simulink model "Senorless"  (R2023a)
settings: Solver=FixedStepDiscrete  StartTime=0.0  StopTime=5  FixedStep=1/FOC_FRQ  RelTol=1e-3
values from neighbouring files (symbols this model uses):
  ADC_REF = 3.6    [Senorless.sldd]
  ADC_SAMPLE_MAX = 32767.0    [Senorless.sldd]
  AMP_GAIN = 16.0    [Senorless.sldd]
  CURR_INPUT = 3276.0    [Senorless.sldd]
  CURR_KI = 380.0    [Senorless.sldd]
  CURR_KP = 0.04    [Senorless.sldd]
  CURR_LIMIT = 0.95    [Senorless.sldd]
  CURR_OVER = 6.0    [Senorless.sldd]
  CURR_POINT_GAIN = 7.0    [Senorless.sldd]
  CURR_STEP = 32760.0    [Senorless.sldd]
  CURR_UNDER = 0.03    [Senorless.sldd]
  CURR_WIDTH = 6552.0    [Senorless.sldd]
  FOC_FRQ = 25000.0    [Senorless.sldd]
  GAMMA = 32767.0    [Senorless.sldd]
  IMAX = 10.0    [Senorless.sldd]
  LPF_FRQ = 2000.0    [Senorless.sldd]
  MOTOR_DAMPER = 2.06E-7    [Senorless.sldd]
  MOTOR_FLUX = 0.00212352    [Senorless.sldd]
  MOTOR_INERTIA = 4.0E-7    [Senorless.sldd]
  MOTOR_LS = 0.000536    [Senorless.sldd]
  MOTOR_PN = 7.0    [Senorless.sldd]
  MOTOR_RS = 4.0    [Senorless.sldd]
  OPEN_IQ = 0.28    [Senorless.sldd]
  OPEN_IQ_MIN = 0.05    [Senorless.sldd]
  OPEN_IQ_SLOW = 0.1    [Senorless.sldd]
  OPEN_SPD = 1000.0    [Senorless.sldd]
  OPEN_SPD_SLOW = 180.0    [Senorless.sldd]
  OPEN_TIME = 0.5    [Senorless.sldd]
  OPEN_TIME_NFO = 0.5    [Senorless.sldd]
  PLL_LIMIT = 0.9    [Senorless.sldd]
  PLL_WIDTH = 800.0    [Senorless.sldd]
  PWM_FRQ = 96000000.0    [Senorless.sldd]
  RS_HUNT = 0.02    [Senorless.sldd]
  SMOK_FRQ = 600.0    [Senorless.sldd]
  SPD_LIMIT = 0.9    [Senorless.sldd]
  SPD_LPF_LEVEL = 0.0    [Senorless.sldd]
  SPD_MAX = 12000.0    [Senorless.sldd]
  SPD_MIN = 4000.0    [Senorless.sldd]
  SPD_REDUCE = 380.0    [Senorless.sldd]
  SPD_STEP = 6.0    [Senorless.sldd]
  SPD_WIDTH = 20.0    [Senorless.sldd]
  THETA_ERR_LIMIT = 8192.0    [Senorless.sldd]
  TS_POINT_GAIN = 10.0    [Senorless.sldd]
  UDC = 48.0    [Senorless.sldd]
  UDC_GAIN = 21.0    [Senorless.sldd]
  UDC_POINT_GAIN = 10.0    [Senorless.sldd]
undefined symbols (not defined in the file or in its folder): curr_q_ki, curr_q_kp, DiscIntNeverNeededParam, magnitude, PLL_LPF_LEVEL, Udc
libraries: simulink x20, slpidlib x5, mcbcontrolslib x2, mcbplantlib x1, autolibpmsmexterior x1, spspowerguiLib x1
(part 2 of 8)

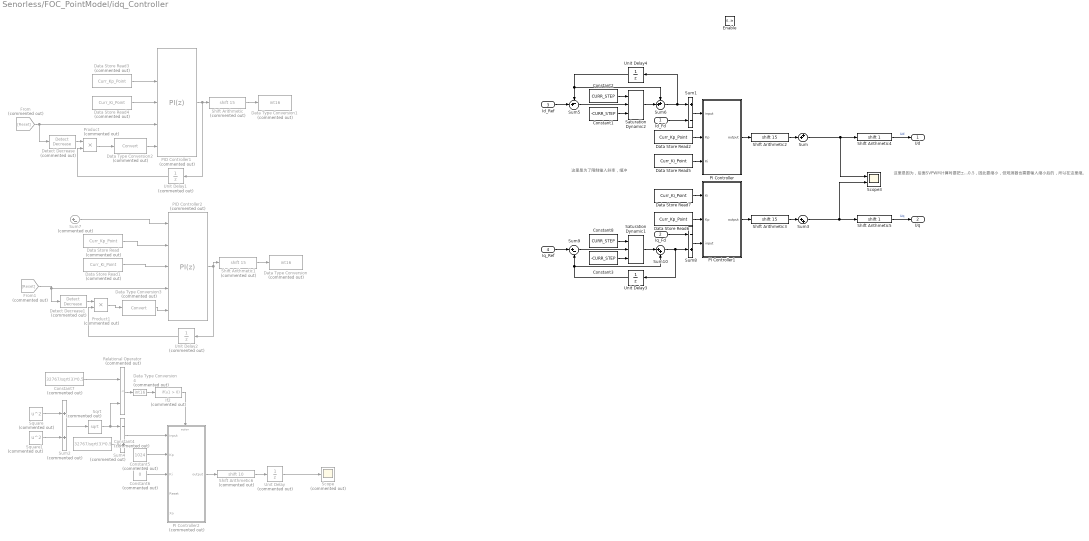
== system Senorless/FOC_PointModel/idq_Controller ==
  note: 这里是为了限制输入斜率，缓冲
  note: 这里是因为，后面SVPWM计算时要把±1映射去±0.5，因此要缩小，但观测器也需要输入缩小后的，所以在这里缩。
  Id_Fd : Inport
  Iq_Fd : Inport  Port=2
  Id_Ref : Inport  Port=3
  Iq_Ref : Inport  Port=4
  Enable : EnablePort  StatesWhenEnabling=reset
  Constant1 : Constant  Value=-CURR_STEP  OutDataTypeStr=int16
  Constant2 : Constant  Value=CURR_STEP  OutDataTypeStr=int16
  Constant3 : Constant  Value=-CURR_STEP  OutDataTypeStr=int16
  Constant4 : Constant  Commented=on  Value=32767/sqrt(3)*0.5  OutDataTypeStr=int32
  Constant5 : Constant  Commented=on  Value=1024  OutDataTypeStr=int16
  Constant6 : Constant  Commented=on  Value=0  OutDataTypeStr=int16
  Constant7 : Constant  Commented=on  Value=32767/sqrt(3)*0.5  OutDataTypeStr=int32
  Constant8 : Constant  Value=CURR_STEP  OutDataTypeStr=int16
  Data Store Read : DataStoreRead  Commented=on  DataStoreName=Curr_Kp_Point  IndexOptions=Index vector (dialog)  Indices=1  OutputSizes=1
  Data Store Read1 : DataStoreRead  Commented=on  DataStoreName=Curr_Ki_Point  IndexOptions=Index vector (dialog)  Indices=1  OutputSizes=1
  Data Store Read2 : DataStoreRead  DataStoreName=Curr_Kp_Point  IndexOptions=Index vector (dialog)  Indices=1  OutputSizes=1
  Data Store Read3 : DataStoreRead  Commented=on  DataStoreName=Curr_Kp_Point  IndexOptions=Index vector (dialog)  Indices=1  OutputSizes=1
  Data Store Read4 : DataStoreRead  Commented=on  DataStoreName=Curr_Ki_Point  IndexOptions=Index vector (dialog)  Indices=1  OutputSizes=1
  Data Store Read5 : DataStoreRead  DataStoreName=Curr_Ki_Point  IndexOptions=Index vector (dialog)  Indices=1  OutputSizes=1
  Data Store Read6 : DataStoreRead  DataStoreName=Curr_Kp_Point  IndexOptions=Index vector (dialog)  Indices=1  OutputSizes=1
  Data Store Read7 : DataStoreRead  DataStoreName=Curr_Ki_Point  IndexOptions=Index vector (dialog)  Indices=1  OutputSizes=1
  Data Type Conversion : DataTypeConversion  Commented=on  OutDataTypeStr=int16  SaturateOnIntegerOverflow=off  RndMeth=Floor
  Data Type Conversion1 : DataTypeConversion  Commented=on  OutDataTypeStr=int16  SaturateOnIntegerOverflow=off  RndMeth=Floor
  Data Type Conversion2 : DataTypeConversion  Commented=on  SaturateOnIntegerOverflow=off  RndMeth=Floor
  Data Type Conversion3 : DataTypeConversion  Commented=on  SaturateOnIntegerOverflow=off  RndMeth=Floor
  Data Type Conversion4 : DataTypeConversion  Commented=on  OutDataTypeStr=int16  SaturateOnIntegerOverflow=off
  Detect Decrease : simulink/Logic and Bit Operations/Detect Decrease  Commented=on  vinit=0.0  OutDataTypeStr=uint8
  Detect Decrease1 : simulink/Logic and Bit Operations/Detect Decrease  Commented=on  vinit=0.0  OutDataTypeStr=uint8
  From : From  Commented=on  GotoTag=Reset
  From1 : From  Commented=on  GotoTag=Reset
  If2 : If  Commented=on  ShowElse=off
  PI Controller : Subsystem
      settings: MinAlgLoopOccurrences=on
  PI Controller1 : Subsystem
      settings: MinAlgLoopOccurrences=on
  PI Controller2 : Subsystem  Commented=on  TreatAsAtomicUnit=on
      settings: MinAlgLoopOccurrences=on
  PID Controller1 : slpidlib/PID Controller  Commented=on  Controller=PI  Form=Parallel  TimeDomain=Discrete-time  UseExternalTs=off  SampleTime=-1  IntegratorMethod=Forward Euler  FilterMethod=Forward Euler  ControllerParametersSource=external  P=curr_q_kp  I=curr_q_ki  UseKiTs=off  D=0  N=100  UseFilter=on  TunerSelectOption=Transfer Function Based (PID Tuner App)  ZeroCross=off  InitialConditionSource=external  InitialConditionForIntegrator=0  InitialConditionForFilter=0  DifferentiatorICPrevScaledInput=0  ExternalReset=either  TrackingMode=off  Kt=1  LimitOutput=on  SatLimitsSource=internal  UpperSaturationLimit=32767*32767  LowerSaturationLimit=-32767*32767  LinearizeAsGain=on  AntiWindupMode=clamping  Kb=1  LimitIntegrator=on  UpperIntegratorSaturationLimit=32767*32767  LowerIntegratorSaturationLimit=-32767*32767  RndMeth=Zero  SaturateOnIntegerOverflow=on  PGainOutDataTypeStr=int32  PProdOutDataTypeStr=int32  POutMin=[]  POutMax=[]  IGainOutDataTypeStr=int32  IProdOutDataTypeStr=int32  IOutMin=[]  IOutMax=[]  DOutMin=[]  DOutMax=[]  NOutMin=[]  NOutMax=[]  SumOutDataTypeStr=int32  SumOutMin=[]  SumOutMax=[]  SaturationOutDataTypeStr=int32  SaturationOutMin=[]  SaturationOutMax=[]  PParamMin=[]  PParamMax=[]  IParamMin=[]  IParamMax=[]  DParamMin=[]  DParamMax=[]  NParamMin=[]  NParamMax=[]  KbParamMin=[]  KbParamMax=[]  KtParamMin=[]  KtParamMax=[]  KbOutMin=[]  KbOutMax=[]  KtOutMin=[]  KtOutMax=[]  IntegratorOutDataTypeStr=int32  IntegratorOutMin=[]  IntegratorOutMax=[]  FilterOutMin=[]  FilterOutMax=[]  SumI1OutMin=[]  SumI1OutMax=[]  SumI2OutMin=[]  SumI2OutMax=[]  SumI3OutMin=[]  SumI3OutMax=[]  SumI4OutMin=[]  SumI4OutMax=[]  SumDOutMin=[]  SumDOutMax=[]  SumAccumDataTypeStr=int32  DifferentiatorOutMin=[]  DifferentiatorOutMax=[]  FilterDiffOutCoefMin=[]  FilterDiffOutCoefMax=[]  ReciprocalOutMin=[]  ReciprocalOutMax=[]  SumDenOutMin=[]  SumDenOutMax=[]  SumNumOutMin=[]  SumNumOutMax=[]  DivideOutMin=[]  DivideOutMax=[]  UdiffTsProdOutMin=[]  UdiffTsProdOutMax=[]  NTsProdOutMin=[]  NTsProdOutMax=[]  UintegralTsProdOutMin=[]  UintegralTsProdOutMax=[]  UngainTsProdOutMin=[]  UngainTsProdOutMax=[]  ClampingZeroOutDataTypeStr=int32  ClampingZeroOutMin=[]  ClampingZeroOutMax=[]  FilterDenConstantOutDataTypeStr=Inherit: Inherit via back propagation  FilterDenConstantOutMin=[]  FilterDenConstantOutMax=[]  PCopyOutDataTypeStr=Inherit: Inherit via back propagation  PCopyOutMin=[]  PCopyOutMax=[]  NCopyOutDataTypeStr=Inherit: Inherit via back propagation  NCopyOutMin=[]  NCopyOutMax=[]  IntegratorContinuousStateAttributes=''  IntegratorStateMustResolveToSignalObject=off  IntegratorRTWStateStorageClass=Auto  FilterContinuousStateAttributes=''  FilterStateMustResolveToSignalObject=off  FilterRTWStateStorageClass=Auto  ParallelPVariant=ExternalParameters  IdealPVariant=Disabled  IVariant=ExternalParameters  DVariant=Disabled  IntegratorVariant=Discrete  SatVariant=Enabled  AWVariant=DiscClampingParallel  PCopyVariant=Disabled  TRVariant=Disabled  FdbkBlocksVariant=Forward  IdealPFdbkVariant=Disabled  SatFdbkVariant=Disabled  DerivativeFilterVariant=Disabled  NVariant=Disabled  NCopyVariant=Disabled_SignalSpec  FilterICVariant=Disabled  IntegratorICVariant=ExternalICs  ExternalResetVariant=ExternalReset  TRSumVariant=Passthrough  SumFdbkVariant=Disabled  SumVariant=Sum_PI  TsampFilterVariant=InternalTs  TsampNgainVariant=Passthrough  TsampIntegralVariant=Disabled_SignalSpec  ExternalSaturationOutDataTypeStr=int32
  PID Controller2 : slpidlib/PID Controller  Commented=on  Controller=PI  Form=Parallel  TimeDomain=Discrete-time  UseExternalTs=off  SampleTime=-1  IntegratorMethod=Forward Euler  FilterMethod=Forward Euler  ControllerParametersSource=external  P=curr_q_kp  I=curr_q_ki  UseKiTs=off  D=0  N=100  UseFilter=on  TunerSelectOption=Transfer Function Based (PID Tuner App)  ZeroCross=off  InitialConditionSource=external  InitialConditionForIntegrator=0  InitialConditionForFilter=0  DifferentiatorICPrevScaledInput=0  ExternalReset=either  TrackingMode=off  Kt=1  LimitOutput=on  SatLimitsSource=internal  UpperSaturationLimit=32767*32767  LowerSaturationLimit=-32767*32767  LinearizeAsGain=on  AntiWindupMode=none  Kb=1  LimitIntegrator=on  UpperIntegratorSaturationLimit=32767*32767  LowerIntegratorSaturationLimit=-32767*32767  RndMeth=Zero  SaturateOnIntegerOverflow=on  PGainOutDataTypeStr=int32  PProdOutDataTypeStr=int32  POutMin=[]  POutMax=[]  IGainOutDataTypeStr=int32  IProdOutDataTypeStr=int32  IOutMin=[]  IOutMax=[]  DOutMin=[]  DOutMax=[]  NOutMin=[]  NOutMax=[]  SumOutDataTypeStr=int32  SumOutMin=[]  SumOutMax=[]  SaturationOutDataTypeStr=int32  SaturationOutMin=[]  SaturationOutMax=[]  PParamMin=[]  PParamMax=[]  IParamMin=[]  IParamMax=[]  DParamMin=[]  DParamMax=[]  NParamMin=[]  NParamMax=[]  KbParamMin=[]  KbParamMax=[]  KtParamMin=[]  KtParamMax=[]  KbOutMin=[]  KbOutMax=[]  KtOutMin=[]  KtOutMax=[]  IntegratorOutDataTypeStr=int32  IntegratorOutMin=[]  IntegratorOutMax=[]  FilterOutMin=[]  FilterOutMax=[]  SumI1OutMin=[]  SumI1OutMax=[]  SumI2OutMin=[]  SumI2OutMax=[]  SumI3OutMin=[]  SumI3OutMax=[]  SumI4OutMin=[]  SumI4OutMax=[]  SumDOutMin=[]  SumDOutMax=[]  SumAccumDataTypeStr=int32  DifferentiatorOutMin=[]  DifferentiatorOutMax=[]  FilterDiffOutCoefMin=[]  FilterDiffOutCoefMax=[]  ReciprocalOutMin=[]  ReciprocalOutMax=[]  SumDenOutMin=[]  SumDenOutMax=[]  SumNumOutMin=[]  SumNumOutMax=[]  DivideOutMin=[]  DivideOutMax=[]  UdiffTsProdOutMin=[]  UdiffTsProdOutMax=[]  NTsProdOutMin=[]  NTsProdOutMax=[]  UintegralTsProdOutMin=[]  UintegralTsProdOutMax=[]  UngainTsProdOutMin=[]  UngainTsProdOutMax=[]  ClampingZeroOutDataTypeStr=int32  ClampingZeroOutMin=[]  ClampingZeroOutMax=[]  FilterDenConstantOutDataTypeStr=Inherit: Inherit via back propagation  FilterDenConstantOutMin=[]  FilterDenConstantOutMax=[]  PCopyOutDataTypeStr=Inherit: Inherit via back propagation  PCopyOutMin=[]  PCopyOutMax=[]  NCopyOutDataTypeStr=Inherit: Inherit via back propagation  NCopyOutMin=[]  NCopyOutMax=[]  IntegratorContinuousStateAttributes=''  IntegratorStateMustResolveToSignalObject=off  IntegratorRTWStateStorageClass=Auto  FilterContinuousStateAttributes=''  FilterStateMustResolveToSignalObject=off  FilterRTWStateStorageClass=Auto  ParallelPVariant=ExternalParameters  IdealPVariant=Disabled  IVariant=ExternalParameters  DVariant=Disabled  IntegratorVariant=Discrete  SatVariant=Enabled  AWVariant=Passthrough  PCopyVariant=Disabled  TRVariant=Disabled  FdbkBlocksVariant=Forward  IdealPFdbkVariant=Disabled  SatFdbkVariant=Disabled  DerivativeFilterVariant=Disabled  NVariant=Disabled  NCopyVariant=Disabled_SignalSpec  FilterICVariant=Disabled  IntegratorICVariant=ExternalICs  ExternalResetVariant=ExternalReset  TRSumVariant=Passthrough  SumFdbkVariant=Disabled  SumVariant=Sum_PI  TsampFilterVariant=InternalTs  TsampNgainVariant=Passthrough  TsampIntegralVariant=Disabled_SignalSpec  ExternalSaturationOutDataTypeStr=int32
  Product : Product  Commented=on  OutDataTypeStr=int32  RndMeth=Zero
  Product1 : Product  Commented=on  OutDataTypeStr=int32  RndMeth=Zero
  Relational Operator : RelationalOperator  Commented=on  Operator=<  OutDataTypeStr=boolean  RndMeth=Zero  InputSameDT=off
  Saturation Dynamic1 : simulink/Discontinuities/Saturation Dynamic  OutMin=[]  OutMax=[]  OutDataTypeStr=Inherit: Same as second input  OutDataType=fixdt(1, 16)  OutScaling=2^-10  RndMeth=Zero  DoSatur=off
  Saturation Dynamic2 : simulink/Discontinuities/Saturation Dynamic  OutMin=[]  OutMax=[]  OutDataTypeStr=Inherit: Same as second input  OutDataType=fixdt(1, 16)  OutScaling=2^-10  RndMeth=Zero  DoSatur=off
  Scope : Scope  Commented=on
  Scope3 : Scope  NumInputPorts=2
  Shift Arithmetic : ArithShift  Commented=on  BitShiftNumber=15
  Shift Arithmetic1 : ArithShift  Commented=on  BitShiftNumber=15
  Shift Arithmetic2 : ArithShift  BitShiftNumber=15
  Shift Arithmetic3 : ArithShift  BitShiftNumber=15
  Shift Arithmetic4 : ArithShift  BitShiftNumber=1
  Shift Arithmetic5 : ArithShift  BitShiftNumber=1
  Shift Arithmetic6 : ArithShift  Commented=on  BitShiftNumber=10
  Sqrt : Sqrt  Commented=on  OutputSignalType=real  RndMeth=Zero
  Square : Math  Commented=on  Operator=square
  Square1 : Math  Commented=on  Operator=square
  Sum : Sum  Inputs=++|
  Sum1 : Sum  Inputs=+-  AccumDataTypeStr=int32  OutDataTypeStr=int32  RndMeth=Zero
  Sum10 : Sum  Inputs=|++  OutDataTypeStr=int16  RndMeth=Zero
  Sum2 : Sum  Commented=on  RndMeth=Zero
  Sum3 : Sum  Inputs=|++
  Sum4 : Sum  Commented=on  Inputs=-+  RndMeth=Zero
  Sum5 : Sum  Inputs=-+|  AccumDataTypeStr=int16  OutDataTypeStr=int16  RndMeth=Zero
  Sum6 : Sum  Inputs=++|  OutDataTypeStr=int16  RndMeth=Zero
  Sum7 : Sum  Commented=on  Inputs=|+-  AccumDataTypeStr=int32  OutDataTypeStr=int32  RndMeth=Zero
  Sum8 : Sum  Inputs=-+  AccumDataTypeStr=int32  OutDataTypeStr=int32  RndMeth=Zero
  Sum9 : Sum  Inputs=|+-  AccumDataTypeStr=int16  OutDataTypeStr=int16  RndMeth=Zero
  Unit Delay : UnitDelay  Commented=on  SampleTime=-1  HasFrameUpgradeWarning=on
  Unit Delay1 : UnitDelay  Commented=on  SampleTime=-1  HasFrameUpgradeWarning=on
  Unit Delay2 : UnitDelay  Commented=on  SampleTime=-1  HasFrameUpgradeWarning=on
  Unit Delay3 : UnitDelay  SampleTime=-1  HasFrameUpgradeWarning=on
  Unit Delay4 : UnitDelay  SampleTime=-1  HasFrameUpgradeWarning=on
  Ud : Outport
  Uq : Outport  Port=2
  wires:
  Sum7/1 -> PID Controller2/1
  Shift Arithmetic/1 -> Data Type Conversion1/1
  Shift Arithmetic1/1 -> Data Type Conversion/1
  Data Store Read/1 -> PID Controller2/2
  Data Store Read1/1 -> PID Controller2/3
  Data Store Read3/1 -> PID Controller1/2
  Data Store Read4/1 -> PID Controller1/3
  PID Controller1/1 -> Unit Delay1/1, Shift Arithmetic/1
  Unit Delay1/1 -> Product/2
  Detect Decrease/1 -> Product/1
  Product/1 -> Data Type Conversion2/1
  From/1 -> PID Controller1/4, Detect Decrease/1
  Unit Delay2/1 -> Product1/2
  Product1/1 -> Data Type Conversion3/1
  From1/1 -> PID Controller2/4, Detect Decrease1/1
  PID Controller2/1 -> Shift Arithmetic1/1, Unit Delay2/1
  Detect Decrease1/1 -> Product1/1
  Data Type Conversion3/1 -> PID Controller2/5
  PI Controller/1(output) -> Shift Arithmetic2/1
  Data Store Read5/1 -> PI Controller/3(Ki)
  Data Type Conversion2/1 -> PID Controller1/5
  Sum1/1 -> PI Controller/1(input)
  PI Controller1/1(output) -> Shift Arithmetic3/1
  Data Store Read2/1 -> PI Controller/2(Kp)
  Saturation Dynamic2/1 -> Sum6/2
  Unit Delay4/1 -> Sum6/1, Sum5/1
  Sum6/1 -> Unit Delay4/1, Sum1/1
  Constant1/1 -> Saturation Dynamic2/3
  Sum3/1 -> Shift Arithmetic5/1, Scope3/2
  Shift Arithmetic3/1 -> Sum3/1
  Sum/1 -> Shift Arithmetic4/1, Scope3/1
  Shift Arithmetic4/1 -> Ud/1  "Ud"
  Shift Arithmetic5/1 -> Uq/1  "Uq"
  Square1/1 -> Sum2/2
  Square/1 -> Sum2/1
  Sum2/1 -> Sqrt/1
  Constant4/1 -> Sum4/2
  Sqrt/1 -> Relational Operator/2, Sum4/1
  Sum4/1 -> PI Controller2/1(input)
  Constant5/1 -> PI Controller2/2(Kp)
  Constant6/1 -> PI Controller2/3(Ki)
  Id_Ref/1 -> Sum5/2
  PI Controller2/1(output) -> Shift Arithmetic6/1
  Unit Delay/1 -> Scope/1
  Constant7/1 -> Relational Operator/1
  Relational Operator/1 -> Data Type Conversion4/1
  If2/1 -> PI Controller2/Action
  Data Type Conversion4/1 -> If2/1
  Shift Arithmetic6/1 -> Unit Delay/1
  Id_Fd/1 -> Sum1/2
  Sum5/1 -> Saturation Dynamic2/2
  Constant2/1 -> Saturation Dynamic2/1
  Sum9/1 -> Saturation Dynamic1/2
  Constant8/1 -> Saturation Dynamic1/1
  Constant3/1 -> Saturation Dynamic1/3
  Data Store Read7/1 -> PI Controller1/1(Ki)
  Data Store Read6/1 -> PI Controller1/2(Kp)
  Sum8/1 -> PI Controller1/3(input)
  Iq_Fd/1 -> Sum8/1
  Saturation Dynamic1/1 -> Sum10/1
  Unit Delay3/1 -> Sum10/2, Sum9/2
  Iq_Ref/1 -> Sum9/1
  Sum10/1 -> Sum8/2, Unit Delay3/1
  Shift Arithmetic2/1 -> Sum/2

== system Senorless/FOC_PointModel/sincos_512 ==
  theta : Inport
  Constant3 : Constant  Value=16384  OutDataTypeStr=uint16
  Shift Arithmetic : ArithShift  BitShiftNumber=7
  Shift Arithmetic1 : ArithShift  BitShiftNumber=7
  Sin : Lookup_n-D  NumberOfTableDimensions=1  BreakpointsSpecification=Even spacing  BreakpointsForDimension1=uint16(linspace(0,511,512))  BreakpointsForDimension1DataTypeStr=uint16  IndexSearchMethod=Linear search  BeginIndexSearchUsingPreviousIndexResult=on  UseOneInputPortForAllInputData=on  Table=int16(32767*sin(linspace(0,2*pi,512)))  TableDataTypeStr=int16  IntermediateResultsDataTypeStr=int32  InterpMethod=Flat  ExtrapMethod=Clip  RemoveProtectionInput=on  ApplyFullPrecisionForLinearInterpolation=on  InternalRulePriority=Speed  OutDataTypeStr=int16  RndMeth=Zero  FractionDataTypeStr=fixdt(1,16,0)  InputSameDT=off
  Sin1 : Lookup_n-D  NumberOfTableDimensions=1  BreakpointsSpecification=Even spacing  BreakpointsForDimension1=uint16(linspace(0,511,512))  BreakpointsForDimension1DataTypeStr=uint16  IndexSearchMethod=Linear search  BeginIndexSearchUsingPreviousIndexResult=on  UseOneInputPortForAllInputData=on  Table=int16(32767*sin(linspace(0,2*pi,512)))  TableDataTypeStr=int16  IntermediateResultsDataTypeStr=int32  InterpMethod=Flat  ExtrapMethod=Clip  RemoveProtectionInput=on  ApplyFullPrecisionForLinearInterpolation=on  InternalRulePriority=Speed  OutDataTypeStr=int16  RndMeth=Zero  FractionDataTypeStr=fixdt(1,16,0)  InputSameDT=off
  Sum2 : Sum  Inputs=|++
  theta1 : InportShadow
  sin : Outport
  cos : Outport  Port=2
  wires:
  Sin1/1 -> cos/1
  Sin/1 -> sin/1
  Shift Arithmetic/1 -> Sin1/1
  Sum2/1 -> Shift Arithmetic/1
  Constant3/1 -> Sum2/2
  Shift Arithmetic1/1 -> Sin/1
  theta1/1 -> Sum2/1
  theta/1 -> Shift Arithmetic1/1

== system Senorless/FOC_PointModel/停止等待 ==
  Action Port : ActionPort  InitializeStates=reset  ActionPortLabel=case [ 0 ]:
  Constant1 : Constant  Value=0  OutDataTypeStr=int16
  Constant2 : Constant  Value=0  OutDataTypeStr=uint16
  Constant3 : Constant  Value=0  OutDataTypeStr=int16
  Theta : Outport
  Iq : Outport  Port=2
  Id : Outport  Port=3
  wires:
  Constant1/1 -> Iq/1
  Constant2/1 -> Theta/1
  Constant3/1 -> Id/1

== system Senorless/FOC_PointModel/切闭环角度差 ==
  Obs_Theta : Inport
  Open_Theta : Inport  Port=2
  Enable : EnablePort  StatesWhenEnabling=reset
  Abs : Abs  RndMeth=Zero  SaturateOnIntegerOverflow=off
  Sum4 : Sum  Inputs=+-  OutDataTypeStr=int32  RndMeth=Zero
  Unit Delay5 : UnitDelay  SampleTime=-1  HasFrameUpgradeWarning=on
  Unit Delay6 : UnitDelay  SampleTime=-1  HasFrameUpgradeWarning=on
  Unit Delay7 : UnitDelay  SampleTime=-1  HasFrameUpgradeWarning=on
  Theta_Rrr : Outport
  +-Err : Outport  Port=2
  wires:
  Unit Delay6/1 -> Sum4/2
  Unit Delay7/1 -> Sum4/1
  Sum4/1 -> Abs/1, +-Err/1
  Unit Delay5/1 -> Unit Delay7/1
  Abs/1 -> Theta_Rrr/1
  Obs_Theta/1 -> Unit Delay5/1
  Open_Theta/1 -> Unit Delay6/1
